simulink model "gm_sampleModel61556_pp_34_1_sub"  (R2023b)
settings: Solver=VariableStepAuto  StartTime=0.0  StopTime=10.0  RelTol=1e-3
libraries: simulink x34
(part 1 of 2)
settings Model: Creator=CW  LastModifiedBy=CW
settings OptimizationCC: BlockReduction=off  ConditionallyExecuteInputs=off
settings DebuggingCC: ArtificialAlgebraicLoopMsg=none  InheritedTsInSrcMsg=none

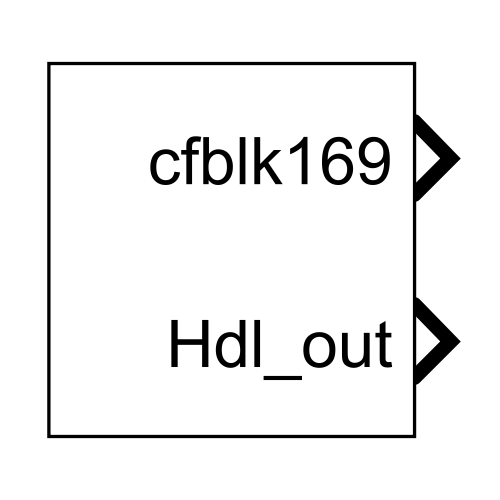
[thumbnail: Simulink's stored preview of the top-level diagram]
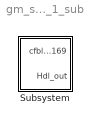
== system gm_sampleModel61556_pp_34_1_sub ==
  Subsystem : Subsystem

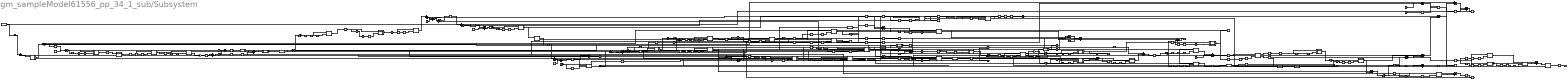
== system gm_sampleModel61556_pp_34_1_sub/Subsystem ==
  Reshape{,1..5} (6 alike) : Reshape
  cfblk1 : Subsystem  mask(Compare To Zero){relop=<=, OutDataTypeStr=uint8, ZeroCross=on}
      mask prompts: relop "Simulink:masks:Operator_MP"; OutDataTypeStr "Simulink:masks:OutputDataType_MP"; ZeroCross "Simulink:masks:EnableZerocrossingDetection_MP"
      mask help: Simulink:masks:CompareToZero_MD
      mask init:
      | OutDataTypeStr = 'uint8';
      | ZeroCross = 'on';
      | blkName = 'sampleModel61556_pp_34_1_sub/Subsystem/cfblk1';
      | relop = '<=';
      | setValue = 'fixdt(0, 8)';
      mask TypeOptions relop: == | ~= | < | <= | >= | >
      mask TypeOptions OutDataTypeStr: Simulink:masks:uint8 | Simulink:masks:boolean
      mask Callback ZeroCross: sl('zeroCrossEnable', gcbh);
      mask Display: disp([relop,' 0'])
  cfblk10 : Subsystem
  cfblk102_inst : Subsystem
  cfblk103 : Subsystem
  cfblk{19,24,26,50,55,57,59,72,104..105,112,115,128,136,138,141,147,158,160} (19 alike) : Sum  OutDataTypeStr=uint8  AccumDataTypeStr=uint8  SampleTime=1
  cfblk{11,30,53,71,81,97,106} (7 alike) : Sum  Inputs=+  OutDataTypeStr=uint8
  cfblk{13,20,22,32,46,82,85,88,107,116,121,134..135,140,154} (15 alike) : Sum  Inputs=+-  OutDataTypeStr=uint8  AccumDataTypeStr=uint8  SampleTime=1
  cfblk{5,15,42,109,123,145..146,162} (8 alike) : Product  Inputs=*/  OutDataTypeStr=uint8  RndMeth=Zero  SaturateOnIntegerOverflow=on  SampleTime=1
  cfblk110 : Subsystem  mask(Real World Value Increment){}
      mask help: Simulink:masks:RealWorldValueIncrement_MD
      mask Display: disp('V++')
  cfblk111 : Subsystem
  cfblk113 : Signum  SampleTime=1
  cfblk{52,80,114,126} (4 alike) : Gain  Gain="fi(0,0,8,7,\"hex\",\"80\")"  ParamDataTypeStr=fixdt(0, 8, 7)  OutDataTypeStr=uint8  SampleTime=1
  cfblk118 : Subsystem
  cfblk119 : Subsystem
  cfblk12 : Subsystem
  cfblk{7,23,25,31,51,63..64,73,87,98,122,142..143,149,152} (15 alike) : MinMax  OutDataTypeStr=uint8
  cfblk{6,41,44,47,60,75,124,132,161,163} (10 alike) : Sum  OutDataTypeStr=uint8  AccumDataTypeStr=uint8  RndMeth=Nearest  SampleTime=1
  cfblk124_const_val : Constant  Value=0  VectorParams1D=off  OutDataTypeStr=uint8  SampleTime=1
  cfblk125 : Subsystem
  cfblk127 : Subsystem
  cfblk129 : Subsystem
  cfblk{17,68,74,99,131,155..156,159} (8 alike) : Abs  SampleTime=1  OutDataTypeStr=uint8  SaturateOnIntegerOverflow=off
  cfblk132_const_val : Constant  Value=0  VectorParams1D=off  OutDataTypeStr=uint8  SampleTime=1
  cfblk133 : Subsystem
  cfblk139 : Subsystem
  cfblk14 : ComplexToRealImag  SampleTime=1
  cfblk144 : Subsystem
  cfblk150 : ComplexToRealImag  SampleTime=1
  cfblk153 : Subsystem
  cfblk157 : Subsystem
  cfblk16 : Subsystem  mask(Real World Value Increment){}
      mask help: Simulink:masks:RealWorldValueIncrement_MD
      mask Display: disp('V++')
  cfblk161_const_val : Constant  Value=0  VectorParams1D=off  OutDataTypeStr=uint8  SampleTime=1
  cfblk163_const_val : Constant  Value=0  VectorParams1D=off  OutDataTypeStr=uint8  SampleTime=1
  cfblk171 : Constant  OutDataTypeStr=uint8  SampleTime=1
  cfblk172 : Constant  OutDataTypeStr=uint8  SampleTime=1
  cfblk173 : Subsystem
  cfblk175 : Subsystem
  cfblk176 : Subsystem
  cfblk177 : Subsystem
  cfblk178 : Subsystem
  cfblk179 : Subsystem
  cfblk180 : Switch  Threshold=double(0)  OutDataTypeStr=uint8  SampleTime=1  SaturateOnIntegerOverflow=off  InputSameDT=off
  cfblk184 : Switch  Threshold=double(0)  OutDataTypeStr=uint8  SampleTime=1  SaturateOnIntegerOverflow=off  InputSameDT=off
  cfblk{186..190,192..197,199..205} (18 alike) : Delay  DelayLength=double(2)  InitialCondition=0  SampleTime=1
  cfblk191 : Subsystem
  cfblk2 : Subsystem  mask(Detect Rise Nonnegative){vinit=double(0), InputProcessing=Elements as channels (sample based), OutDataTypeStr=uint8}
      mask prompts: vinit "Simulink:masks:InitialCondition_MP"; InputProcessing "Simulink:masks:InputProcessing_MP"; OutDataTypeStr "Simulink:masks:OutputDataType_MP"
      mask help: Simulink:masks:DetectRiseNonnegative_MD
      mask init:
      | InputProcessing = 'Elements as channels (sample based)';
      | OutDataTypeStr = 'uint8';
      | vinit = double(0);
      mask TypeOptions InputProcessing: Simulink:masks:ColumnsAsChannelsFrameBased | Simulink:masks:ElementsAsChannelsSampleBased
      mask TypeOptions OutDataTypeStr: Simulink:masks:uint8 | Simulink:masks:boolean
      mask Display: fprintf('U >= 0\n&  NOT\nU/z >= 0')
  cfblk{206..207,209..210,213..215} (7 alike) : DataTypeConversion  OutDataTypeStr=fixdt(0,8,0)
  cfblk208 : Subsystem
  cfblk21 : Subsystem
  cfblk211 : Subsystem
  cfblk212 : Subsystem
  cfblk3 : Subsystem
  cfblk35 : Subsystem
  cfblk36 : Subsystem
  cfblk37 : Subsystem
  cfblk38 : Subsystem  mask(Real World Value Increment){}
      mask help: Simulink:masks:RealWorldValueIncrement_MD
      mask Display: disp('V++')
  cfblk39 : ComplexToRealImag  SampleTime=1
  cfblk4 : Subsystem
  cfblk41_const_val : Constant  Value=0  VectorParams1D=off  OutDataTypeStr=uint8  SampleTime=1
  cfblk43_inst : Subsystem
  cfblk44_const_val : Constant  Value=0  VectorParams1D=off  OutDataTypeStr=uint8  SampleTime=1
  cfblk47_const_val : Constant  Value=0  VectorParams1D=off  OutDataTypeStr=uint8  SampleTime=1
  cfblk49 : Subsystem
  cfblk54 : Subsystem
  cfblk60_const_val : Constant  Value=0  VectorParams1D=off  OutDataTypeStr=uint8  SampleTime=1
  cfblk61_const_val : Constant  Value=double(0)  VectorParams1D=off  OutDataTypeStr=double  SampleTime=1
  cfblk62 : Signum  SampleTime=1
  cfblk65 : Subsystem
  cfblk66 : Subsystem  mask(Real World Value Increment){}
      mask help: Simulink:masks:RealWorldValueIncrement_MD
      mask Display: disp('V++')
  cfblk67 : Subsystem  mask(Real World Value Increment){}
      mask help: Simulink:masks:RealWorldValueIncrement_MD
      mask Display: disp('V++')
  cfblk6_const_val : Constant  Value=0  VectorParams1D=off  OutDataTypeStr=uint8  SampleTime=1
  cfblk70_inst : Subsystem
  cfblk75_const_val : Constant  Value=0  VectorParams1D=off  OutDataTypeStr=uint8  SampleTime=1
  cfblk78 : Subsystem
  cfblk8 : Subsystem
  cfblk83 : Subsystem
  cfblk84_inst : Subsystem
  cfblk86 : Subsystem
  cfblk9 : Subsystem
  cfblk90_inst : Subsystem
  cfblk91 : Subsystem
  cfblk93_inst : Subsystem
  cfblk96 : Subsystem
  compare{,1..3,6,9,14..15,21..24,26,28,32} (15 alike) : simulink/Logic and Bit Operations/Compare To Constant  relop=>=  const=255  OutDataTypeStr=boolean
  compare{4..5,7..8,10..13,16..20,25,27,29..31,33} (19 alike) : simulink/Logic and Bit Operations/Compare To Constant  relop=>=  const=0  OutDataTypeStr=boolean
  emi_{6,22,30,38,46,55,63,79,87,96,104,112,120,128,136,144,152,160,168,176,184,192,200,225,233,241,249,257,266,274,282,298,306,314} (34 alike) : DataTypeConversion  OutDataTypeStr=fixdt(0,8,0)
  emi_{7,31,39,88,105,113,121,129,153,177,226,234,283,299,307} (15 alike) : Delay  DelayLength=double(2)  InitialCondition=255  SampleTime=1
  emi_{23,47,56,64,80,97,137,145,161,169,185,193,201,242,250,258,267,275,315} (19 alike) : Delay  DelayLength=double(2)  InitialCondition=0  SampleTime=1
  cfblk169 : Outport  OutDataTypeStr=uint8  SampleTime=1  InitialOutput=[0]  VectorParamsAs1DForOutWhenUnconnected=off
  Hdl_out : Outport  Port=2  OutDataTypeStr=uint8  SampleTime=1
  wires:
  cfblk1/1(y) -> Reshape1/1
  cfblk10/1(emi_2) -> cfblk66/1(u)
  cfblk102_inst/1(out1) -> cfblk180/2
  cfblk103/1(emi_18) -> cfblk15/1
  cfblk104/1 -> emi_113/1, cfblk144/1(emi_107)
  cfblk105/1 -> cfblk32/2, cfblk115/2
  cfblk106/1 -> emi_121/1, cfblk191/1(emi_115)
  cfblk107/1 -> cfblk31/1
  cfblk109/1 -> cfblk93_inst/1(in1)
  cfblk11/1 -> Reshape5/1
  cfblk110/1(y) -> cfblk46/1, cfblk197/1
  cfblk111/1(emi_26) -> cfblk82/1, cfblk67/1(u)
  cfblk112/1 -> cfblk206/1
  cfblk113/1 -> cfblk126/1
  cfblk114/1 -> cfblk214/1
  cfblk115/1 -> cfblk80/1
  cfblk116/1 -> cfblk41/1
  cfblk118/1(emi_42) -> cfblk5/2, cfblk71/1
  cfblk119/1(emi_50) -> cfblk158/2
  cfblk119/2(emi_51) -> cfblk6/1
  cfblk12/1(emi_59) -> cfblk150/1, cfblk134/2
  cfblk121/1 -> cfblk109/2, cfblk11/1
  cfblk122/1 -> cfblk154/2
  cfblk123/1 -> cfblk81/1
  cfblk124/1 -> cfblk107/1, emi_315/1, cfblk96/1(emi_309)
  cfblk125/1(emi_75) -> cfblk209/1
  cfblk126/1 -> cfblk134/1
  cfblk127/1(emi_83) -> cfblk25/1
  cfblk128/1 -> cfblk121/1
  cfblk129/1(emi_91) -> cfblk210/1
  cfblk129/2(emi_92) -> cfblk14/1
  cfblk13/1 -> emi_226/1, cfblk49/1(emi_219)
  cfblk131/1 -> cfblk16/1(u)
  cfblk132/1 -> emi_234/1, cfblk212/1(emi_228)
  cfblk133/1(emi_148) -> emi_299/1, cfblk9/1(emi_293), cfblk23/1
  cfblk134/1 -> cfblk26/1
  cfblk135/1 -> cfblk116/2
  cfblk136/1 -> cfblk147/1
  cfblk138/1 -> cfblk154/1
  cfblk139/1(emi_100) -> cfblk138/2, cfblk179/1(In1)
  cfblk14/1 -> cfblk160/2
  cfblk14/2 -> cfblk175/1(In1)
  cfblk140/1 -> cfblk138/1, emi_169/1, cfblk3/1(emi_163)
  cfblk141/1 -> cfblk24/1, cfblk200/1
  cfblk142/1 -> cfblk20/1
  cfblk143/1 -> emi_161/1, cfblk211/1(emi_155)
  cfblk144/1(emi_108) -> cfblk55/1
  cfblk145/1 -> emi_275/1, emi_193/1, cfblk83/1(emi_269), cfblk37/1(emi_187)
  cfblk146/1 -> cfblk141/1, cfblk102_inst/1(in1)
  cfblk147/1 -> cfblk202/1
  Reshape/1 -> cfblk84_inst/1(in1)
  cfblk149/1 -> cfblk104/1
  cfblk15/1 -> cfblk99/1
  cfblk150/1 -> cfblk64/1
  cfblk150/2 -> Reshape3/1, cfblk97/1
  cfblk152/1 -> cfblk57/1
  cfblk153/1(emi_124) -> cfblk194/1, cfblk193/1
  cfblk154/1 -> cfblk135/1, cfblk51/1
  cfblk155/1 -> cfblk57/2
  cfblk156/1 -> emi_88/1, cfblk127/1(emi_82)
  cfblk157/1(emi_34) -> emi_283/1, cfblk86/1(emi_277)
  cfblk158/1 -> cfblk142/1
  cfblk159/1 -> cfblk195/1, cfblk42/2
  cfblk16/1(y) -> cfblk155/1
  cfblk160/1 -> cfblk105/2, cfblk145/1
  cfblk161/1 -> cfblk146/2
  cfblk162/1 -> emi_105/1, cfblk139/1(emi_99)
  cfblk163/1 -> cfblk173/1(In1)
  cfblk17/1 -> emi_47/1, cfblk118/1(emi_41)
  cfblk171/1 -> cfblk7/1
  cfblk172/1 -> cfblk26/2
  cfblk173/1(Out1) -> cfblk178/1(In1), cfblk42/1
  cfblk175/1(Out1) -> cfblk2/1(U)
  cfblk176/1(Out1) -> cfblk113/1, cfblk190/1
  cfblk177/1(Out1) -> cfblk75/1
  cfblk178/1(Out1) -> cfblk46/2
  cfblk179/1(Out1) -> cfblk149/1
  cfblk180/1 -> cfblk85/1
  cfblk184/1 -> cfblk136/1, cfblk53/1
  cfblk186/1 -> cfblk109/1
  cfblk187/1 -> cfblk135/2
  cfblk188/1 -> cfblk59/1
  cfblk189/1 -> cfblk128/1
  cfblk19/1 -> cfblk73/1
  cfblk190/1 -> cfblk162/2
  cfblk191/1(emi_116) -> cfblk140/2
  cfblk192/1 -> cfblk93_inst/2(in2)
  cfblk193/1 -> cfblk184/1
  cfblk194/1 -> cfblk180/3
  cfblk195/1 -> cfblk121/2
  cfblk196/1 -> cfblk19/1
  cfblk197/1 -> cfblk184/3
  cfblk199/1 -> cfblk22/2
  cfblk2/1(Y) -> cfblk180/1
  cfblk20/1 -> cfblk177/1(In1)
  cfblk200/1 -> cfblk84_inst/2(in2)
  cfblk201/1 -> cfblk146/1
  cfblk202/1 -> cfblk1/1(u)
  cfblk203/1 -> cfblk85/2
  cfblk204/1 -> cfblk88/1
  cfblk205/1 -> cfblk43_inst/2(in2)
  cfblk206/1 -> cfblk199/1
  cfblk207/1 -> cfblk112/1
  cfblk208/1(emi_132) -> cfblk112/2
  cfblk209/1 -> emi_201/1, cfblk205/1, cfblk4/1(emi_195)
  cfblk21/1(emi_140) -> cfblk59/2, cfblk131/1
  cfblk210/1 -> emi_80/1, cfblk125/1(emi_74)
  cfblk211/1(emi_156) -> cfblk88/2
  cfblk212/1(emi_229) -> cfblk143/1
  cfblk213/1 -> cfblk44/1, cfblk207/1
  cfblk214/1 -> cfblk72/1
  cfblk215/1 -> cfblk72/2
  cfblk22/1 -> cfblk43_inst/1(in1)
  cfblk23/1 -> emi_31/1, cfblk111/1(emi_25)
  cfblk24/1 -> cfblk60/1
  cfblk25/1 -> emi_39/1, cfblk157/1(emi_33)
  cfblk26/1 -> cfblk70_inst/2(in2)
  cfblk3/1(emi_164) -> cfblk19/2, cfblk13/2
  cfblk30/1 -> cfblk20/2
  cfblk31/1 -> cfblk39/1, emi_137/1, cfblk208/1(emi_131)
  cfblk32/1 -> cfblk136/2, cfblk201/1
  Reshape1/1 -> cfblk22/1
  cfblk35/1(emi_172) -> cfblk70_inst/1(in1), cfblk15/2
  cfblk36/1(emi_180) -> emi_267/1, cfblk8/1(emi_260)
  cfblk37/1(emi_188) -> emi_242/1, cfblk54/1(emi_236)
  cfblk38/1(y) -> cfblk163/1
  cfblk39/1 -> cfblk160/1
  cfblk39/2 -> cfblk152/1
  cfblk4/1(emi_196) -> cfblk107/2, cfblk105/1
  cfblk41/1 -> cfblk158/1, Hdl_out/1
  cfblk42/1 -> cfblk196/1
  cfblk43_inst/1(out1) -> cfblk184/2
  cfblk44/1 -> Reshape4/1
  cfblk46/1 -> cfblk156/1
  cfblk47/1 -> cfblk123/1
  cfblk49/1(emi_220) -> cfblk62/1
  cfblk49/2(emi_221) -> cfblk52/1
  cfblk5/1 -> cfblk55/2, emi_129/1, cfblk153/1(emi_123)
  cfblk50/1 -> cfblk90_inst/1(in1)
  cfblk51/1 -> emi_153/1, cfblk133/1(emi_147)
  cfblk52/1 -> cfblk17/1
  cfblk53/1 -> cfblk124/1
  cfblk54/1(emi_237) -> cfblk50/2
  cfblk55/1 -> cfblk186/1
  cfblk57/1 -> cfblk87/1
  Reshape2/1 -> cfblk169/1
  cfblk59/1 -> cfblk161/1
  cfblk6/1 -> cfblk82/2, emi_97/1, cfblk129/1(emi_90)
  cfblk60/1 -> emi_307/1, cfblk91/1(emi_301)
  cfblk62/1 -> cfblk176/1(In1), cfblk106/1
  cfblk63/1 -> cfblk204/1
  cfblk64/1 -> cfblk32/1, cfblk104/2, emi_250/1, cfblk65/1(emi_244)
  cfblk65/1(emi_245) -> cfblk90_inst/2(in2), emi_23/1, cfblk103/1(emi_17), cfblk30/1
  cfblk66/1(y) -> cfblk159/1
  cfblk67/1(y) -> cfblk110/1(u)
  cfblk68/1 -> emi_56/1, emi_145/1, cfblk21/1(emi_139), cfblk119/1(emi_49), cfblk5/1
  cfblk7/1 -> cfblk123/2
  cfblk70_inst/1(out1) -> cfblk188/1
  cfblk71/1 -> cfblk192/1
  cfblk72/1 -> cfblk213/1
  cfblk73/1 -> cfblk68/1
  cfblk74/1 -> emi_177/1, cfblk35/1(emi_171)
  cfblk75/1 -> cfblk74/1
  cfblk78/1(emi_253) -> cfblk215/1
  Reshape3/1 -> cfblk203/1
  cfblk8/1(emi_261) -> cfblk140/1
  cfblk8/2(emi_262) -> cfblk114/1
  cfblk80/1 -> cfblk132/1, cfblk162/1
  cfblk81/1 -> cfblk147/2
  cfblk82/1 -> cfblk24/2, emi_7/1, cfblk10/1(emi_1)
  cfblk83/1(emi_270) -> cfblk50/1
  cfblk84_inst/1(out1) -> emi_185/1, cfblk36/1(emi_179)
  cfblk85/1 -> cfblk128/2
  cfblk86/1(emi_278) -> cfblk116/1
  cfblk87/1 -> cfblk145/2
  cfblk88/1 -> emi_64/1, emi_258/1, cfblk78/1(emi_252), cfblk12/1(emi_58)
  cfblk9/1(emi_294) -> cfblk189/1
  cfblk90_inst/1(out1) -> Reshape2/1
  cfblk91/1(emi_302) -> cfblk13/1
  Reshape4/1 -> cfblk141/2, cfblk38/1(u)
  cfblk93_inst/1(out1) -> cfblk115/1
  Reshape5/1 -> cfblk47/1
  cfblk96/1(emi_310) -> Reshape/1
  cfblk97/1 -> cfblk63/1
  cfblk98/1 -> cfblk102_inst/2(in2)
  cfblk99/1 -> cfblk187/1
  emi_104/1 -> compare/1
  emi_105/1 -> emi_104/1
  emi_112/1 -> compare1/1
  emi_113/1 -> emi_112/1
  emi_120/1 -> compare2/1
  emi_121/1 -> emi_120/1
  emi_128/1 -> compare3/1
  emi_129/1 -> emi_128/1
  emi_136/1 -> compare4/1
  emi_137/1 -> emi_136/1
  emi_144/1 -> compare5/1
  emi_145/1 -> emi_144/1
  emi_152/1 -> compare6/1
  emi_153/1 -> emi_152/1
  emi_160/1 -> compare7/1
  emi_161/1 -> emi_160/1
  emi_168/1 -> compare8/1
  emi_169/1 -> emi_168/1
  emi_176/1 -> compare9/1
  emi_177/1 -> emi_176/1
  emi_184/1 -> compare10/1
  emi_185/1 -> emi_184/1
  emi_192/1 -> compare11/1
  emi_193/1 -> emi_192/1
  emi_200/1 -> compare12/1
  emi_201/1 -> emi_200/1
  emi_22/1 -> compare13/1
  emi_225/1 -> compare14/1
  emi_226/1 -> emi_225/1
  emi_23/1 -> emi_22/1
  emi_233/1 -> compare15/1
  emi_234/1 -> emi_233/1
  emi_241/1 -> compare16/1
  emi_242/1 -> emi_241/1
  emi_249/1 -> compare17/1
  emi_250/1 -> emi_249/1
  emi_257/1 -> compare18/1
  emi_258/1 -> emi_257/1
  emi_266/1 -> compare19/1
  emi_267/1 -> emi_266/1
  emi_274/1 -> compare20/1
  emi_275/1 -> emi_274/1
  emi_282/1 -> compare21/1
  emi_283/1 -> emi_282/1
  emi_298/1 -> compare23/1
  emi_299/1 -> emi_298/1
  emi_30/1 -> compare22/1
  emi_306/1 -> compare24/1
  emi_307/1 -> emi_306/1
  emi_31/1 -> emi_30/1
  emi_314/1 -> compare25/1
  emi_315/1 -> emi_314/1
  emi_38/1 -> compare26/1
  emi_39/1 -> emi_38/1
  emi_46/1 -> compare27/1
  emi_47/1 -> emi_46/1
  emi_55/1 -> compare29/1
  emi_56/1 -> emi_55/1
  emi_6/1 -> compare28/1
  emi_63/1 -> compare30/1
  emi_64/1 -> emi_63/1
  emi_7/1 -> emi_6/1
  emi_79/1 -> compare31/1
  emi_80/1 -> emi_79/1
  emi_87/1 -> compare32/1
  emi_88/1 -> emi_87/1
  emi_96/1 -> compare33/1
  emi_97/1 -> emi_96/1
  cfblk124_const_val/1 -> cfblk124/2
  cfblk132_const_val/1 -> cfblk132/2
  cfblk161_const_val/1 -> cfblk161/2
  cfblk163_const_val/1 -> cfblk163/2
  cfblk41_const_val/1 -> cfblk41/2
  cfblk44_const_val/1 -> cfblk44/2
  cfblk47_const_val/1 -> cfblk47/2
  cfblk6_const_val/1 -> cfblk6/2
  cfblk60_const_val/1 -> cfblk60/2
  cfblk61_const_val/1 -> cfblk98/1, cfblk122/1
  cfblk75_const_val/1 -> cfblk75/2
  compare/1 -> cfblk139/2(Action Port)
  compare1/1 -> cfblk144/2(Action Port)
  compare2/1 -> cfblk191/2(Action Port)
  compare3/1 -> cfblk153/2(Action Port)
  compare4/1 -> cfblk208/2(Action Port)
  compare5/1 -> cfblk21/2(Action Port)
  compare6/1 -> cfblk133/2(Action Port)
  compare7/1 -> cfblk211/2(Action Port)
  compare8/1 -> cfblk3/2(Action Port)
  compare9/1 -> cfblk35/2(Action Port)
  compare10/1 -> cfblk36/2(Action Port)
  compare11/1 -> cfblk37/2(Action Port)
  compare12/1 -> cfblk4/2(Action Port)
  compare13/1 -> cfblk103/2(Action Port)
  compare14/1 -> cfblk49/2(Action Port)
  compare15/1 -> cfblk212/2(Action Port)
  compare16/1 -> cfblk54/2(Action Port)
  compare17/1 -> cfblk65/2(Action Port)
  compare18/1 -> cfblk78/2(Action Port)
  compare19/1 -> cfblk8/2(Action Port)
  compare20/1 -> cfblk83/2(Action Port)
  compare21/1 -> cfblk86/2(Action Port)
  compare22/1 -> cfblk111/2(Action Port)
  compare23/1 -> cfblk9/2(Action Port)
  compare24/1 -> cfblk91/2(Action Port)
  compare25/1 -> cfblk96/2(Action Port)
  compare26/1 -> cfblk157/2(Action Port)
  compare27/1 -> cfblk118/2(Action Port)
  compare28/1 -> cfblk10/2(Action Port)
  compare29/1 -> cfblk119/2(Action Port)
  compare30/1 -> cfblk12/2(Action Port)
  compare31/1 -> cfblk125/2(Action Port)
  compare32/1 -> cfblk127/2(Action Port)
  compare33/1 -> cfblk129/2(Action Port)

== system gm_sampleModel61556_pp_34_1_sub/Subsystem/cfblk1 ==
  u : Inport  OutDataTypeStr=uint8  SampleTime=1
  Compare : RelationalOperator  Operator=<=  OutDataTypeStr=fixdt(0, 8)
  Constant : Constant  DisableCoverage=on  Value=0  OutDataTypeStr=Inherit: Inherit via back propagation  SampleTime=-1  PreserveConstantTs=on
  y : Outport  SampleTime=1
  wires:
  u/1 -> Compare/1
  Compare/1 -> y/1
  Constant/1 -> Compare/2

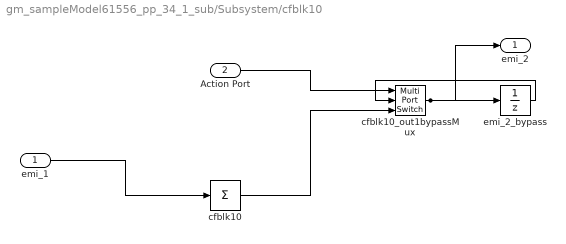
== system gm_sampleModel61556_pp_34_1_sub/Subsystem/cfblk10 ==
  emi_1 : Inport  OutDataTypeStr=uint8  PortDimensions=1  SampleTime=1
  Action Port : Inport  Port=2  OutDataTypeStr=boolean  SampleTime=1
  cfblk10 : Sum  Inputs=+
  cfblk10_out1bypassMux : MultiPortSwitch  DataPortOrder=Zero-based contiguous  Inputs=2  zeroidx=on  OutDataTypeStr=uint8  SampleTime=1  SaturateOnIntegerOverflow=off  InputSameDT=off
  emi_2_bypass : UnitDelay  InitialCondition="fi(0,0,8,0,\"hex\",\"00\")"  SampleTime=1
  emi_2 : Outport  SampleTime=1  InitialOutput=0
  wires:
  Action Port/1 -> cfblk10_out1bypassMux/1
  emi_1/1 -> cfblk10/1
  cfblk10/1 -> cfblk10_out1bypassMux/3
  cfblk10_out1bypassMux/1 -> emi_2_bypass/1, emi_2/1
  emi_2_bypass/1 -> cfblk10_out1bypassMux/2

== system gm_sampleModel61556_pp_34_1_sub/Subsystem/cfblk102_inst ==
  in1 : Inport  OutDataTypeStr=uint8  SampleTime=1
  in2 : Inport  Port=2  OutDataTypeStr=uint8  SampleTime=1
  mul_cfblk102_dotp_mulcomp : Product  Inputs=**  OutDataTypeStr=uint8  SampleTime=1
  out1 : Outport  OutDataTypeStr=uint8  SampleTime=1
  wires:
  in1/1 -> mul_cfblk102_dotp_mulcomp/1
  in2/1 -> mul_cfblk102_dotp_mulcomp/2
  mul_cfblk102_dotp_mulcomp/1 -> out1/1

== system gm_sampleModel61556_pp_34_1_sub/Subsystem/cfblk103 ==
  emi_17 : Inport  OutDataTypeStr=uint8  PortDimensions=1  SampleTime=1
  Action Port : Inport  Port=2  OutDataTypeStr=boolean  SampleTime=1
  cfblk103 : Abs  SampleTime=1  OutDataTypeStr=uint8  SaturateOnIntegerOverflow=off
  cfblk103_out1bypassMux : MultiPortSwitch  DataPortOrder=Zero-based contiguous  Inputs=2  zeroidx=on  OutDataTypeStr=uint8  SampleTime=1  SaturateOnIntegerOverflow=off  InputSameDT=off
  emi_18_bypass : UnitDelay  InitialCondition="fi(0,0,8,0,\"hex\",\"00\")"  SampleTime=1
  emi_18 : Outport  SampleTime=1  InitialOutput=0
  wires:
  Action Port/1 -> cfblk103_out1bypassMux/1
  emi_17/1 -> cfblk103/1
  cfblk103/1 -> cfblk103_out1bypassMux/3
  cfblk103_out1bypassMux/1 -> emi_18_bypass/1, emi_18/1
  emi_18_bypass/1 -> cfblk103_out1bypassMux/2

== system gm_sampleModel61556_pp_34_1_sub/Subsystem/cfblk110 ==
  u : Inport  OutDataTypeStr=uint8  SampleTime=1
  FixPt Constant : Constant  DisableCoverage=on  OutDataTypeStr=Inherit: Inherit via back propagation  SampleTime=-1
  FixPt Data Type Duplicate : DataTypeDuplicate  DisableCoverage=on  NumInputPorts=3
  FixPt Sum1 : Sum  OutDataTypeStr=Inherit: Inherit via back propagation  InputSameDT=on  LockScale=on
  y : Outport  SampleTime=1
  wires:
  u/1 -> FixPt Sum1/1, FixPt Data Type Duplicate/2
  FixPt Constant/1 -> FixPt Sum1/2, FixPt Data Type Duplicate/3
  FixPt Sum1/1 -> FixPt Data Type Duplicate/1, y/1

== system gm_sampleModel61556_pp_34_1_sub/Subsystem/cfblk111 ==
  emi_25 : Inport  OutDataTypeStr=uint8  PortDimensions=1  SampleTime=1
  Action Port : Inport  Port=2  OutDataTypeStr=boolean  SampleTime=1
  cfblk111 : Subsystem  mask(Real World Value Increment){}
      mask help: Simulink:masks:RealWorldValueIncrement_MD
      mask Display: disp('V++')
  cfblk111_out1bypassMux : MultiPortSwitch  DataPortOrder=Zero-based contiguous  Inputs=2  zeroidx=on  OutDataTypeStr=uint8  SampleTime=1  SaturateOnIntegerOverflow=off  InputSameDT=off
  emi_26_bypass : UnitDelay  InitialCondition="fi(0,0,8,0,\"hex\",\"00\")"  SampleTime=1
  emi_26 : Outport  SampleTime=1  InitialOutput=0
  wires:
  Action Port/1 -> cfblk111_out1bypassMux/1
  emi_25/1 -> cfblk111/1(u)
  cfblk111/1(y) -> cfblk111_out1bypassMux/3
  cfblk111_out1bypassMux/1 -> emi_26_bypass/1, emi_26/1
  emi_26_bypass/1 -> cfblk111_out1bypassMux/2

== system gm_sampleModel61556_pp_34_1_sub/Subsystem/cfblk118 ==
  emi_41 : Inport  OutDataTypeStr=uint8  PortDimensions=1  SampleTime=1
  Action Port : Inport  Port=2  OutDataTypeStr=boolean  SampleTime=1
  cfblk118 : MinMax
  cfblk118_out1bypassMux : MultiPortSwitch  DataPortOrder=Zero-based contiguous  Inputs=2  zeroidx=on  OutDataTypeStr=uint8  SampleTime=1  SaturateOnIntegerOverflow=off  InputSameDT=off
  emi_42_bypass : UnitDelay  InitialCondition="fi(0,0,8,0,\"hex\",\"00\")"  SampleTime=1
  emi_42 : Outport  SampleTime=1  InitialOutput=0
  wires:
  Action Port/1 -> cfblk118_out1bypassMux/1
  emi_41/1 -> cfblk118/1
  cfblk118/1 -> cfblk118_out1bypassMux/3
  cfblk118_out1bypassMux/1 -> emi_42_bypass/1, emi_42/1
  emi_42_bypass/1 -> cfblk118_out1bypassMux/2

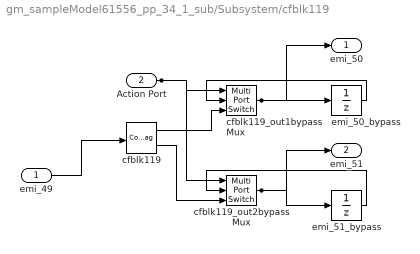
== system gm_sampleModel61556_pp_34_1_sub/Subsystem/cfblk119 ==
  emi_49 : Inport  OutDataTypeStr=uint8  PortDimensions=1  SampleTime=1
  Action Port : Inport  Port=2  OutDataTypeStr=boolean  SampleTime=1
  cfblk119 : ComplexToRealImag  SampleTime=1
  cfblk119_out1bypassMux : MultiPortSwitch  DataPortOrder=Zero-based contiguous  Inputs=2  zeroidx=on  OutDataTypeStr=uint8  SampleTime=1  SaturateOnIntegerOverflow=off  InputSameDT=off
  cfblk119_out2bypassMux : MultiPortSwitch  DataPortOrder=Zero-based contiguous  Inputs=2  zeroidx=on  OutDataTypeStr=uint8  SampleTime=1  SaturateOnIntegerOverflow=off  InputSameDT=off
  emi_50_bypass : UnitDelay  InitialCondition="fi(0,0,8,0,\"hex\",\"00\")"  SampleTime=1
  emi_51_bypass : UnitDelay  InitialCondition="fi(0,0,8,0,\"hex\",\"00\")"  SampleTime=1
  emi_50 : Outport  SampleTime=1  InitialOutput=0
  emi_51 : Outport  Port=2  SampleTime=1  InitialOutput=0
  wires:
  Action Port/1 -> cfblk119_out2bypassMux/1, cfblk119_out1bypassMux/1
  emi_49/1 -> cfblk119/1
  cfblk119/1 -> cfblk119_out1bypassMux/3
  cfblk119/2 -> cfblk119_out2bypassMux/3
  cfblk119_out1bypassMux/1 -> emi_50_bypass/1, emi_50/1
  emi_50_bypass/1 -> cfblk119_out1bypassMux/2
  cfblk119_out2bypassMux/1 -> emi_51_bypass/1, emi_51/1
  emi_51_bypass/1 -> cfblk119_out2bypassMux/2

== system gm_sampleModel61556_pp_34_1_sub/Subsystem/cfblk12 ==
  emi_58 : Inport  OutDataTypeStr=uint8  PortDimensions=1  SampleTime=1
  Action Port : Inport  Port=2  OutDataTypeStr=boolean  SampleTime=1
  cfblk12 : Sum  Inputs=+
  cfblk12_out1bypassMux : MultiPortSwitch  DataPortOrder=Zero-based contiguous  Inputs=2  zeroidx=on  OutDataTypeStr=uint8  SampleTime=1  SaturateOnIntegerOverflow=off  InputSameDT=off
  emi_59_bypass : UnitDelay  InitialCondition="fi(0,0,8,0,\"hex\",\"00\")"  SampleTime=1
  emi_59 : Outport  SampleTime=1  InitialOutput=0
  wires:
  Action Port/1 -> cfblk12_out1bypassMux/1
  emi_58/1 -> cfblk12/1
  cfblk12/1 -> cfblk12_out1bypassMux/3
  cfblk12_out1bypassMux/1 -> emi_59_bypass/1, emi_59/1
  emi_59_bypass/1 -> cfblk12_out1bypassMux/2

== system gm_sampleModel61556_pp_34_1_sub/Subsystem/cfblk125 ==
  emi_74 : Inport  OutDataTypeStr=uint8  PortDimensions=1  SampleTime=1
  Action Port : Inport  Port=2  OutDataTypeStr=boolean  SampleTime=1
  cfblk125 : MinMax
  cfblk125_out1bypassMux : MultiPortSwitch  DataPortOrder=Zero-based contiguous  Inputs=2  zeroidx=on  OutDataTypeStr=uint8  SampleTime=1  SaturateOnIntegerOverflow=off  InputSameDT=off
  emi_75_bypass : UnitDelay  InitialCondition="fi(0,0,8,0,\"hex\",\"00\")"  SampleTime=1
  emi_75 : Outport  SampleTime=1  InitialOutput=0
  wires:
  Action Port/1 -> cfblk125_out1bypassMux/1
  emi_74/1 -> cfblk125/1
  cfblk125/1 -> cfblk125_out1bypassMux/3
  cfblk125_out1bypassMux/1 -> emi_75_bypass/1, emi_75/1
  emi_75_bypass/1 -> cfblk125_out1bypassMux/2

== system gm_sampleModel61556_pp_34_1_sub/Subsystem/cfblk127 ==
  emi_82 : Inport  OutDataTypeStr=uint8  PortDimensions=1  SampleTime=1
  Action Port : Inport  Port=2  OutDataTypeStr=boolean  SampleTime=1
  cfblk127 : MinMax
  cfblk127_out1bypassMux : MultiPortSwitch  DataPortOrder=Zero-based contiguous  Inputs=2  zeroidx=on  OutDataTypeStr=uint8  SampleTime=1  SaturateOnIntegerOverflow=off  InputSameDT=off
  emi_83_bypass : UnitDelay  InitialCondition="fi(0,0,8,0,\"hex\",\"00\")"  SampleTime=1
  emi_83 : Outport  SampleTime=1  InitialOutput=0
  wires:
  Action Port/1 -> cfblk127_out1bypassMux/1
  emi_82/1 -> cfblk127/1
  cfblk127/1 -> cfblk127_out1bypassMux/3
  cfblk127_out1bypassMux/1 -> emi_83_bypass/1, emi_83/1
  emi_83_bypass/1 -> cfblk127_out1bypassMux/2

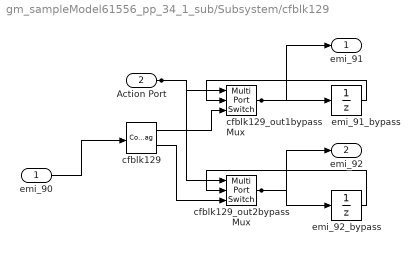
== system gm_sampleModel61556_pp_34_1_sub/Subsystem/cfblk129 ==
  emi_90 : Inport  OutDataTypeStr=uint8  PortDimensions=1  SampleTime=1
  Action Port : Inport  Port=2  OutDataTypeStr=boolean  SampleTime=1
  cfblk129 : ComplexToRealImag  SampleTime=1
  cfblk129_out1bypassMux : MultiPortSwitch  DataPortOrder=Zero-based contiguous  Inputs=2  zeroidx=on  OutDataTypeStr=uint8  SampleTime=1  SaturateOnIntegerOverflow=off  InputSameDT=off
  cfblk129_out2bypassMux : MultiPortSwitch  DataPortOrder=Zero-based contiguous  Inputs=2  zeroidx=on  OutDataTypeStr=uint8  SampleTime=1  SaturateOnIntegerOverflow=off  InputSameDT=off
  emi_91_bypass : UnitDelay  InitialCondition="fi(0,0,8,0,\"hex\",\"00\")"  SampleTime=1
  emi_92_bypass : UnitDelay  InitialCondition="fi(0,0,8,0,\"hex\",\"00\")"  SampleTime=1
  emi_91 : Outport  SampleTime=1  InitialOutput=0
  emi_92 : Outport  Port=2  SampleTime=1  InitialOutput=0
  wires:
  Action Port/1 -> cfblk129_out2bypassMux/1, cfblk129_out1bypassMux/1
  emi_90/1 -> cfblk129/1
  cfblk129/1 -> cfblk129_out1bypassMux/3
  cfblk129/2 -> cfblk129_out2bypassMux/3
  cfblk129_out1bypassMux/1 -> emi_91_bypass/1, emi_91/1
  emi_91_bypass/1 -> cfblk129_out1bypassMux/2
  cfblk129_out2bypassMux/1 -> emi_92_bypass/1, emi_92/1
  emi_92_bypass/1 -> cfblk129_out2bypassMux/2

== system gm_sampleModel61556_pp_34_1_sub/Subsystem/cfblk133 ==
  emi_147 : Inport  OutDataTypeStr=uint8  PortDimensions=1  SampleTime=1
  Action Port : Inport  Port=2  OutDataTypeStr=boolean  SampleTime=1
  Reshape : Reshape
  cfblk133_out1bypassMux : MultiPortSwitch  DataPortOrder=Zero-based contiguous  Inputs=2  zeroidx=on  OutDataTypeStr=uint8  SampleTime=1  SaturateOnIntegerOverflow=off  InputSameDT=off
  emi_148_bypass : UnitDelay  InitialCondition="fi(0,0,8,0,\"hex\",\"00\")"  SampleTime=1
  emi_148 : Outport  SampleTime=1  InitialOutput=0
  wires:
  Action Port/1 -> cfblk133_out1bypassMux/1
  emi_147/1 -> Reshape/1
  Reshape/1 -> cfblk133_out1bypassMux/3
  cfblk133_out1bypassMux/1 -> emi_148_bypass/1, emi_148/1
  emi_148_bypass/1 -> cfblk133_out1bypassMux/2

== system gm_sampleModel61556_pp_34_1_sub/Subsystem/cfblk139 ==
  emi_99 : Inport  OutDataTypeStr=uint8  PortDimensions=1  SampleTime=1
  Action Port : Inport  Port=2  OutDataTypeStr=boolean  SampleTime=1
  Reshape : Reshape
  cfblk139_out1bypassMux : MultiPortSwitch  DataPortOrder=Zero-based contiguous  Inputs=2  zeroidx=on  OutDataTypeStr=uint8  SampleTime=1  SaturateOnIntegerOverflow=off  InputSameDT=off
  emi_100_bypass : UnitDelay  InitialCondition="fi(0,0,8,0,\"hex\",\"00\")"  SampleTime=1
  emi_100 : Outport  SampleTime=1  InitialOutput=0
  wires:
  Action Port/1 -> cfblk139_out1bypassMux/1
  emi_99/1 -> Reshape/1
  Reshape/1 -> cfblk139_out1bypassMux/3
  cfblk139_out1bypassMux/1 -> emi_100_bypass/1, emi_100/1
  emi_100_bypass/1 -> cfblk139_out1bypassMux/2

== system gm_sampleModel61556_pp_34_1_sub/Subsystem/cfblk144 ==
  emi_107 : Inport  OutDataTypeStr=uint8  PortDimensions=1  SampleTime=1
  Action Port : Inport  Port=2  OutDataTypeStr=boolean  SampleTime=1
  cfblk144 : Abs  SampleTime=1  OutDataTypeStr=uint8  SaturateOnIntegerOverflow=off
  cfblk144_out1bypassMux : MultiPortSwitch  DataPortOrder=Zero-based contiguous  Inputs=2  zeroidx=on  OutDataTypeStr=uint8  SampleTime=1  SaturateOnIntegerOverflow=off  InputSameDT=off
  emi_108_bypass : UnitDelay  InitialCondition="fi(0,0,8,0,\"hex\",\"00\")"  SampleTime=1
  emi_108 : Outport  SampleTime=1  InitialOutput=0
  wires:
  Action Port/1 -> cfblk144_out1bypassMux/1
  emi_107/1 -> cfblk144/1
  cfblk144/1 -> cfblk144_out1bypassMux/3
  cfblk144_out1bypassMux/1 -> emi_108_bypass/1, emi_108/1
  emi_108_bypass/1 -> cfblk144_out1bypassMux/2

== system gm_sampleModel61556_pp_34_1_sub/Subsystem/cfblk153 ==
  emi_123 : Inport  OutDataTypeStr=uint8  PortDimensions=1  SampleTime=1
  Action Port : Inport  Port=2  OutDataTypeStr=boolean  SampleTime=1
  cfblk153 : Subsystem  mask(Real World Value Increment){}
      mask help: Simulink:masks:RealWorldValueIncrement_MD
      mask Display: disp('V++')
  cfblk153_out1bypassMux : MultiPortSwitch  DataPortOrder=Zero-based contiguous  Inputs=2  zeroidx=on  OutDataTypeStr=uint8  SampleTime=1  SaturateOnIntegerOverflow=off  InputSameDT=off
  emi_124_bypass : UnitDelay  InitialCondition="fi(0,0,8,0,\"hex\",\"00\")"  SampleTime=1
  emi_124 : Outport  SampleTime=1  InitialOutput=0
  wires:
  Action Port/1 -> cfblk153_out1bypassMux/1
  emi_123/1 -> cfblk153/1(u)
  cfblk153/1(y) -> cfblk153_out1bypassMux/3
  cfblk153_out1bypassMux/1 -> emi_124_bypass/1, emi_124/1
  emi_124_bypass/1 -> cfblk153_out1bypassMux/2

== system gm_sampleModel61556_pp_34_1_sub/Subsystem/cfblk157 ==
  emi_33 : Inport  OutDataTypeStr=uint8  PortDimensions=1  SampleTime=1
  Action Port : Inport  Port=2  OutDataTypeStr=boolean  SampleTime=1
  cfblk157 : Abs  SampleTime=1  OutDataTypeStr=uint8  SaturateOnIntegerOverflow=off
  cfblk157_out1bypassMux : MultiPortSwitch  DataPortOrder=Zero-based contiguous  Inputs=2  zeroidx=on  OutDataTypeStr=uint8  SampleTime=1  SaturateOnIntegerOverflow=off  InputSameDT=off
  emi_34_bypass : UnitDelay  InitialCondition="fi(0,0,8,0,\"hex\",\"00\")"  SampleTime=1
  emi_34 : Outport  SampleTime=1  InitialOutput=0
  wires:
  Action Port/1 -> cfblk157_out1bypassMux/1
  emi_33/1 -> cfblk157/1
  cfblk157/1 -> cfblk157_out1bypassMux/3
  cfblk157_out1bypassMux/1 -> emi_34_bypass/1, emi_34/1
  emi_34_bypass/1 -> cfblk157_out1bypassMux/2

== system gm_sampleModel61556_pp_34_1_sub/Subsystem/cfblk16 ==
  u : Inport  OutDataTypeStr=uint8  SampleTime=1
  FixPt Constant : Constant  DisableCoverage=on  OutDataTypeStr=Inherit: Inherit via back propagation  SampleTime=-1
  FixPt Data Type Duplicate : DataTypeDuplicate  DisableCoverage=on  NumInputPorts=3
  FixPt Sum1 : Sum  OutDataTypeStr=Inherit: Inherit via back propagation  InputSameDT=on  LockScale=on
  y : Outport  SampleTime=1
  wires:
  u/1 -> FixPt Sum1/1, FixPt Data Type Duplicate/2
  FixPt Constant/1 -> FixPt Sum1/2, FixPt Data Type Duplicate/3
  FixPt Sum1/1 -> FixPt Data Type Duplicate/1, y/1

== system gm_sampleModel61556_pp_34_1_sub/Subsystem/cfblk173 ==
  In1 : Inport  OutDataTypeStr=uint8  PortDimensions=1  SampleTime=1
  Out1 : Outport  SampleTime=1  InitialOutput=[0]
  wires:
  In1/1 -> Out1/1

== system gm_sampleModel61556_pp_34_1_sub/Subsystem/cfblk175 ==
  In1 : Inport  OutDataTypeStr=uint8  PortDimensions=1  SampleTime=1
  Out1 : Outport  SampleTime=1  InitialOutput=[0]
  wires:
  In1/1 -> Out1/1

== system gm_sampleModel61556_pp_34_1_sub/Subsystem/cfblk176 ==
  In1 : Inport  OutDataTypeStr=uint8  PortDimensions=1  SampleTime=1
  Out1 : Outport  SampleTime=1  InitialOutput=[0]
  wires:
  In1/1 -> Out1/1

== system gm_sampleModel61556_pp_34_1_sub/Subsystem/cfblk177 ==
  In1 : Inport  OutDataTypeStr=uint8  PortDimensions=1  SampleTime=1
  Out1 : Outport  SampleTime=1  InitialOutput=[0]
  wires:
  In1/1 -> Out1/1

== system gm_sampleModel61556_pp_34_1_sub/Subsystem/cfblk178 ==
  In1 : Inport  OutDataTypeStr=uint8  PortDimensions=1  SampleTime=1
  Out1 : Outport  SampleTime=1  InitialOutput=[0]
  wires:
  In1/1 -> Out1/1

== system gm_sampleModel61556_pp_34_1_sub/Subsystem/cfblk179 ==
  In1 : Inport  OutDataTypeStr=uint8  PortDimensions=1  SampleTime=1
  Out1 : Outport  SampleTime=1  InitialOutput=[0]
  wires:
  In1/1 -> Out1/1

== system gm_sampleModel61556_pp_34_1_sub/Subsystem/cfblk191 ==
  emi_115 : Inport  OutDataTypeStr=uint8  PortDimensions=1  SampleTime=1
  Action Port : Inport  Port=2  OutDataTypeStr=boolean  SampleTime=1
  cfblk191 : Subsystem
      settings: MinAlgLoopOccurrences=on
  emi_116 : Outport  SampleTime=1  InitialOutput=0
  wires:
  Action Port/1 -> cfblk191/Enable
  emi_115/1 -> cfblk191/1(in0)
  cfblk191/1(out0) -> emi_116/1

== system gm_sampleModel61556_pp_34_1_sub/Subsystem/cfblk2 ==
  note: U(k)
  note: Edge
  U : Inport  OutDataTypeStr=uint8  SampleTime=1
  Delay Input1 : UnitDelay  Description=Store in Global RAM  DisableCoverage=on  InitialCondition=vinit  SampleTime=-1  HasFrameUpgradeWarning=on
  FixPt Relational Operator : RelationalOperator  Operator=>  OutDataTypeStr=fixdt(0, 8)  ZeroCross=off  InputSameDT=off
  Nonnegative : Subsystem  mask(Compare To Zero){relop=>=, OutDataTypeStr=boolean, ZeroCross=off}
      mask prompts: relop "Simulink:masks:Operator_MP"; OutDataTypeStr "Simulink:masks:OutputDataType_MP"; ZeroCross "Simulink:masks:EnableZerocrossingDetection_MP"
      mask help: Simulink:masks:CompareToZero_MD
      mask init:
      | OutDataTypeStr = 'boolean';
      | ZeroCross = 'off';
      | blkName = 'sampleModel61556_pp_34_1_sub/Subsystem/cfblk2/Nonnegative';
      | relop = '>=';
      | setValue = 'boolean';
      mask TypeOptions relop: == | ~= | < | <= | >= | >
      mask TypeOptions OutDataTypeStr: Simulink:masks:uint8 | Simulink:masks:boolean
      mask Callback ZeroCross: sl('zeroCrossEnable', gcbh);
      mask Display: disp([relop,' 0'])
  Y : Outport  SampleTime=1
  wires:
  U/1 -> Nonnegative/1(u)
  Delay Input1/1 -> FixPt Relational Operator/2
  FixPt Relational Operator/1 -> Y/1
  Nonnegative/1(y) -> FixPt Relational Operator/1, Delay Input1/1

== system gm_sampleModel61556_pp_34_1_sub/Subsystem/cfblk208 ==
  emi_131 : Inport  OutDataTypeStr=uint8  PortDimensions=1  SampleTime=1
  Action Port : Inport  Port=2  OutDataTypeStr=boolean  SampleTime=1
  cfblk208 : DataTypeConversion  OutDataTypeStr=fixdt(0,8,0)
  cfblk208_out1bypassMux : MultiPortSwitch  DataPortOrder=Zero-based contiguous  Inputs=2  zeroidx=on  OutDataTypeStr=uint8  SampleTime=1  SaturateOnIntegerOverflow=off  InputSameDT=off
  emi_132_bypass : UnitDelay  InitialCondition="fi(0,0,8,0,\"hex\",\"00\")"  SampleTime=1
  emi_132 : Outport  SampleTime=1  InitialOutput=0
  wires:
  Action Port/1 -> cfblk208_out1bypassMux/1
  emi_131/1 -> cfblk208/1
  cfblk208/1 -> cfblk208_out1bypassMux/3
  cfblk208_out1bypassMux/1 -> emi_132_bypass/1, emi_132/1
  emi_132_bypass/1 -> cfblk208_out1bypassMux/2

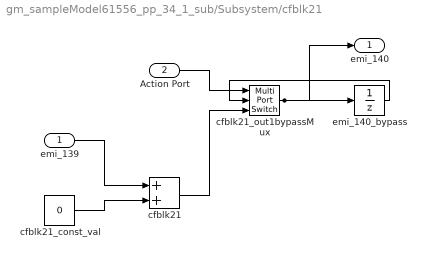
== system gm_sampleModel61556_pp_34_1_sub/Subsystem/cfblk21 ==
  emi_139 : Inport  OutDataTypeStr=uint8  PortDimensions=1  SampleTime=1
  Action Port : Inport  Port=2  OutDataTypeStr=boolean  SampleTime=1
  cfblk21 : Sum  OutDataTypeStr=uint8  AccumDataTypeStr=uint8  RndMeth=Nearest  SampleTime=1
  cfblk21_const_val : Constant  Value=0  VectorParams1D=off  OutDataTypeStr=uint8  SampleTime=1
  cfblk21_out1bypassMux : MultiPortSwitch  DataPortOrder=Zero-based contiguous  Inputs=2  zeroidx=on  OutDataTypeStr=uint8  SampleTime=1  SaturateOnIntegerOverflow=off  InputSameDT=off
  emi_140_bypass : UnitDelay  InitialCondition="fi(0,0,8,0,\"hex\",\"00\")"  SampleTime=1
  emi_140 : Outport  SampleTime=1  InitialOutput=0
  wires:
  Action Port/1 -> cfblk21_out1bypassMux/1
  emi_139/1 -> cfblk21/1
  cfblk21/1 -> cfblk21_out1bypassMux/3
  cfblk21_out1bypassMux/1 -> emi_140_bypass/1, emi_140/1
  emi_140_bypass/1 -> cfblk21_out1bypassMux/2
  cfblk21_const_val/1 -> cfblk21/2

== system gm_sampleModel61556_pp_34_1_sub/Subsystem/cfblk211 ==
  emi_155 : Inport  OutDataTypeStr=uint8  PortDimensions=1  SampleTime=1
  Action Port : Inport  Port=2  OutDataTypeStr=boolean  SampleTime=1
  cfblk211 : DataTypeConversion  OutDataTypeStr=fixdt(0,8,0)
  cfblk211_out1bypassMux : MultiPortSwitch  DataPortOrder=Zero-based contiguous  Inputs=2  zeroidx=on  OutDataTypeStr=uint8  SampleTime=1  SaturateOnIntegerOverflow=off  InputSameDT=off
  emi_156_bypass : UnitDelay  InitialCondition="fi(0,0,8,0,\"hex\",\"00\")"  SampleTime=1
  emi_156 : Outport  SampleTime=1  InitialOutput=0
  wires:
  Action Port/1 -> cfblk211_out1bypassMux/1
  emi_155/1 -> cfblk211/1
  cfblk211/1 -> cfblk211_out1bypassMux/3
  cfblk211_out1bypassMux/1 -> emi_156_bypass/1, emi_156/1
  emi_156_bypass/1 -> cfblk211_out1bypassMux/2

== system gm_sampleModel61556_pp_34_1_sub/Subsystem/cfblk212 ==
  emi_228 : Inport  OutDataTypeStr=uint8  PortDimensions=1  SampleTime=1
  Action Port : Inport  Port=2  OutDataTypeStr=boolean  SampleTime=1
  cfblk212 : DataTypeConversion  OutDataTypeStr=fixdt(0,8,0)
  cfblk212_out1bypassMux : MultiPortSwitch  DataPortOrder=Zero-based contiguous  Inputs=2  zeroidx=on  OutDataTypeStr=uint8  SampleTime=1  SaturateOnIntegerOverflow=off  InputSameDT=off
  emi_229_bypass : UnitDelay  InitialCondition="fi(0,0,8,0,\"hex\",\"00\")"  SampleTime=1
  emi_229 : Outport  SampleTime=1  InitialOutput=0
  wires:
  Action Port/1 -> cfblk212_out1bypassMux/1
  emi_228/1 -> cfblk212/1
  cfblk212/1 -> cfblk212_out1bypassMux/3
  cfblk212_out1bypassMux/1 -> emi_229_bypass/1, emi_229/1
  emi_229_bypass/1 -> cfblk212_out1bypassMux/2

== system gm_sampleModel61556_pp_34_1_sub/Subsystem/cfblk3 ==
  emi_163 : Inport  OutDataTypeStr=uint8  PortDimensions=1  SampleTime=1
  Action Port : Inport  Port=2  OutDataTypeStr=boolean  SampleTime=1
  cfblk3 : Constant  Value=0  OutDataTypeStr=uint8  SampleTime=1
  cfblk3_out1bypassMux : MultiPortSwitch  DataPortOrder=Zero-based contiguous  Inputs=2  zeroidx=on  OutDataTypeStr=uint8  SampleTime=1  SaturateOnIntegerOverflow=off  InputSameDT=off
  emi_164_bypass : UnitDelay  InitialCondition="fi(0,0,8,0,\"hex\",\"00\")"  SampleTime=1
  emi_164 : Outport  SampleTime=1  InitialOutput=0
  wires:
  Action Port/1 -> cfblk3_out1bypassMux/1
  cfblk3/1 -> cfblk3_out1bypassMux/3
  cfblk3_out1bypassMux/1 -> emi_164_bypass/1, emi_164/1
  emi_164_bypass/1 -> cfblk3_out1bypassMux/2

== system gm_sampleModel61556_pp_34_1_sub/Subsystem/cfblk35 ==
  emi_171 : Inport  OutDataTypeStr=uint8  PortDimensions=1  SampleTime=1
  Action Port : Inport  Port=2  OutDataTypeStr=boolean  SampleTime=1
  cfblk35 : Abs  SampleTime=1  OutDataTypeStr=uint8  SaturateOnIntegerOverflow=off
  cfblk35_out1bypassMux : MultiPortSwitch  DataPortOrder=Zero-based contiguous  Inputs=2  zeroidx=on  OutDataTypeStr=uint8  SampleTime=1  SaturateOnIntegerOverflow=off  InputSameDT=off
  emi_172_bypass : UnitDelay  InitialCondition="fi(0,0,8,0,\"hex\",\"00\")"  SampleTime=1
  emi_172 : Outport  SampleTime=1  InitialOutput=0
  wires:
  Action Port/1 -> cfblk35_out1bypassMux/1
  emi_171/1 -> cfblk35/1
  cfblk35/1 -> cfblk35_out1bypassMux/3
  cfblk35_out1bypassMux/1 -> emi_172_bypass/1, emi_172/1
  emi_172_bypass/1 -> cfblk35_out1bypassMux/2

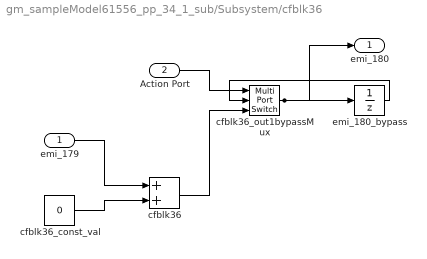
== system gm_sampleModel61556_pp_34_1_sub/Subsystem/cfblk36 ==
  emi_179 : Inport  OutDataTypeStr=uint8  PortDimensions=1  SampleTime=1
  Action Port : Inport  Port=2  OutDataTypeStr=boolean  SampleTime=1
  cfblk36 : Sum  OutDataTypeStr=uint8  AccumDataTypeStr=uint8  RndMeth=Nearest  SampleTime=1
  cfblk36_const_val : Constant  Value=0  VectorParams1D=off  OutDataTypeStr=uint8  SampleTime=1
  cfblk36_out1bypassMux : MultiPortSwitch  DataPortOrder=Zero-based contiguous  Inputs=2  zeroidx=on  OutDataTypeStr=uint8  SampleTime=1  SaturateOnIntegerOverflow=off  InputSameDT=off
  emi_180_bypass : UnitDelay  InitialCondition="fi(0,0,8,0,\"hex\",\"00\")"  SampleTime=1
  emi_180 : Outport  SampleTime=1  InitialOutput=0
  wires:
  Action Port/1 -> cfblk36_out1bypassMux/1
  emi_179/1 -> cfblk36/1
  cfblk36/1 -> cfblk36_out1bypassMux/3
  cfblk36_out1bypassMux/1 -> emi_180_bypass/1, emi_180/1
  emi_180_bypass/1 -> cfblk36_out1bypassMux/2
  cfblk36_const_val/1 -> cfblk36/2

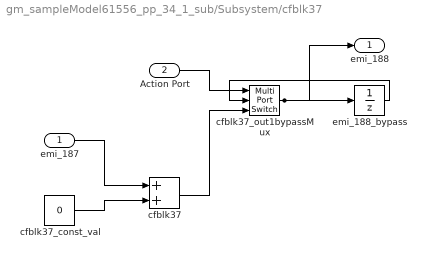
== system gm_sampleModel61556_pp_34_1_sub/Subsystem/cfblk37 ==
  emi_187 : Inport  OutDataTypeStr=uint8  PortDimensions=1  SampleTime=1
  Action Port : Inport  Port=2  OutDataTypeStr=boolean  SampleTime=1
  cfblk37 : Sum  OutDataTypeStr=uint8  AccumDataTypeStr=uint8  RndMeth=Nearest  SampleTime=1
  cfblk37_const_val : Constant  Value=0  VectorParams1D=off  OutDataTypeStr=uint8  SampleTime=1
  cfblk37_out1bypassMux : MultiPortSwitch  DataPortOrder=Zero-based contiguous  Inputs=2  zeroidx=on  OutDataTypeStr=uint8  SampleTime=1  SaturateOnIntegerOverflow=off  InputSameDT=off
  emi_188_bypass : UnitDelay  InitialCondition="fi(0,0,8,0,\"hex\",\"00\")"  SampleTime=1
  emi_188 : Outport  SampleTime=1  InitialOutput=0
  wires:
  Action Port/1 -> cfblk37_out1bypassMux/1
  emi_187/1 -> cfblk37/1
  cfblk37/1 -> cfblk37_out1bypassMux/3
  cfblk37_out1bypassMux/1 -> emi_188_bypass/1, emi_188/1
  emi_188_bypass/1 -> cfblk37_out1bypassMux/2
  cfblk37_const_val/1 -> cfblk37/2

== system gm_sampleModel61556_pp_34_1_sub/Subsystem/cfblk38 ==
  u : Inport  OutDataTypeStr=uint8  SampleTime=1
  FixPt Constant : Constant  DisableCoverage=on  OutDataTypeStr=Inherit: Inherit via back propagation  SampleTime=-1
  FixPt Data Type Duplicate : DataTypeDuplicate  DisableCoverage=on  NumInputPorts=3
  FixPt Sum1 : Sum  OutDataTypeStr=Inherit: Inherit via back propagation  InputSameDT=on  LockScale=on
  y : Outport  SampleTime=1
  wires:
  u/1 -> FixPt Sum1/1, FixPt Data Type Duplicate/2
  FixPt Constant/1 -> FixPt Sum1/2, FixPt Data Type Duplicate/3
  FixPt Sum1/1 -> FixPt Data Type Duplicate/1, y/1

== system gm_sampleModel61556_pp_34_1_sub/Subsystem/cfblk4 ==
  emi_195 : Inport  OutDataTypeStr=uint8  PortDimensions=1  SampleTime=1
  Action Port : Inport  Port=2  OutDataTypeStr=boolean  SampleTime=1
  cfblk4 : Subsystem  mask(Detect Rise Positive){vinit=double(0), InputProcessing=Elements as channels (sample based), OutDataTypeStr=uint8}
      mask prompts: vinit "Simulink:masks:InitialCondition_MP"; InputProcessing "Simulink:masks:InputProcessing_MP"; OutDataTypeStr "Simulink:masks:OutputDataType_MP"
      mask help: Simulink:masks:DetectRisePositive_MD
      mask TypeOptions InputProcessing: Simulink:masks:ColumnsAsChannelsFrameBased | Simulink:masks:ElementsAsChannelsSampleBased
      mask TypeOptions OutDataTypeStr: Simulink:masks:uint8 | Simulink:masks:boolean
      mask Display: fprintf('U > 0\n&  NOT\nU/z > 0')
  cfblk4_out1bypassMux : MultiPortSwitch  DataPortOrder=Zero-based contiguous  Inputs=2  zeroidx=on  OutDataTypeStr=uint8  SampleTime=1  SaturateOnIntegerOverflow=off  InputSameDT=off
  emi_196_bypass : UnitDelay  InitialCondition="fi(0,0,8,0,\"hex\",\"00\")"  SampleTime=1
  emi_196 : Outport  SampleTime=1  InitialOutput=0
  wires:
  Action Port/1 -> cfblk4_out1bypassMux/1, cfblk4/2(Action Port_out2)
  emi_195/1 -> cfblk4/1(U)
  cfblk4/1(Y) -> cfblk4_out1bypassMux/3
  cfblk4_out1bypassMux/1 -> emi_196_bypass/1, emi_196/1
  emi_196_bypass/1 -> cfblk4_out1bypassMux/2

== system gm_sampleModel61556_pp_34_1_sub/Subsystem/cfblk43_inst ==
  in1 : Inport  OutDataTypeStr=uint8  SampleTime=1
  in2 : Inport  Port=2  OutDataTypeStr=uint8  SampleTime=1
  mul_cfblk43_dotp_mulcomp : Product  Inputs=**  OutDataTypeStr=uint8  SampleTime=1
  out1 : Outport  OutDataTypeStr=uint8  SampleTime=1
  wires:
  in1/1 -> mul_cfblk43_dotp_mulcomp/1
  in2/1 -> mul_cfblk43_dotp_mulcomp/2
  mul_cfblk43_dotp_mulcomp/1 -> out1/1

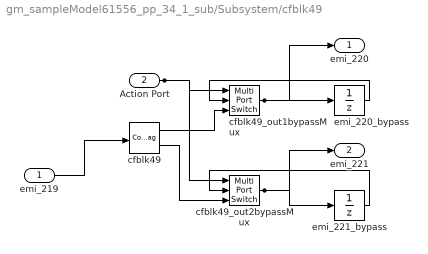
== system gm_sampleModel61556_pp_34_1_sub/Subsystem/cfblk49 ==
  emi_219 : Inport  OutDataTypeStr=uint8  PortDimensions=1  SampleTime=1
  Action Port : Inport  Port=2  OutDataTypeStr=boolean  SampleTime=1
  cfblk49 : ComplexToRealImag  SampleTime=1
  cfblk49_out1bypassMux : MultiPortSwitch  DataPortOrder=Zero-based contiguous  Inputs=2  zeroidx=on  OutDataTypeStr=uint8  SampleTime=1  SaturateOnIntegerOverflow=off  InputSameDT=off
  cfblk49_out2bypassMux : MultiPortSwitch  DataPortOrder=Zero-based contiguous  Inputs=2  zeroidx=on  OutDataTypeStr=uint8  SampleTime=1  SaturateOnIntegerOverflow=off  InputSameDT=off
  emi_220_bypass : UnitDelay  InitialCondition="fi(0,0,8,0,\"hex\",\"00\")"  SampleTime=1
  emi_221_bypass : UnitDelay  InitialCondition="fi(0,0,8,0,\"hex\",\"00\")"  SampleTime=1
  emi_220 : Outport  SampleTime=1  InitialOutput=0
  emi_221 : Outport  Port=2  SampleTime=1  InitialOutput=0
  wires:
  Action Port/1 -> cfblk49_out2bypassMux/1, cfblk49_out1bypassMux/1
  emi_219/1 -> cfblk49/1
  cfblk49/1 -> cfblk49_out1bypassMux/3
  cfblk49/2 -> cfblk49_out2bypassMux/3
  cfblk49_out1bypassMux/1 -> emi_220_bypass/1, emi_220/1
  emi_220_bypass/1 -> cfblk49_out1bypassMux/2
  cfblk49_out2bypassMux/1 -> emi_221_bypass/1, emi_221/1
  emi_221_bypass/1 -> cfblk49_out2bypassMux/2

== system gm_sampleModel61556_pp_34_1_sub/Subsystem/cfblk54 ==
  emi_236 : Inport  OutDataTypeStr=uint8  PortDimensions=1  SampleTime=1
  Action Port : Inport  Port=2  OutDataTypeStr=boolean  SampleTime=1
  cfblk54 : Sum  Inputs=+
  cfblk54_out1bypassMux : MultiPortSwitch  DataPortOrder=Zero-based contiguous  Inputs=2  zeroidx=on  OutDataTypeStr=uint8  SampleTime=1  SaturateOnIntegerOverflow=off  InputSameDT=off
  emi_237_bypass : UnitDelay  InitialCondition="fi(0,0,8,0,\"hex\",\"00\")"  SampleTime=1
  emi_237 : Outport  SampleTime=1  InitialOutput=0
  wires:
  Action Port/1 -> cfblk54_out1bypassMux/1
  emi_236/1 -> cfblk54/1
  cfblk54/1 -> cfblk54_out1bypassMux/3
  cfblk54_out1bypassMux/1 -> emi_237_bypass/1, emi_237/1
  emi_237_bypass/1 -> cfblk54_out1bypassMux/2

== system gm_sampleModel61556_pp_34_1_sub/Subsystem/cfblk65 ==
  emi_244 : Inport  OutDataTypeStr=uint8  PortDimensions=1  SampleTime=1
  Action Port : Inport  Port=2  OutDataTypeStr=boolean  SampleTime=1
  cfblk65 : Sum  Inputs=+
  cfblk65_out1bypassMux : MultiPortSwitch  DataPortOrder=Zero-based contiguous  Inputs=2  zeroidx=on  OutDataTypeStr=uint8  SampleTime=1  SaturateOnIntegerOverflow=off  InputSameDT=off
  emi_245_bypass : UnitDelay  InitialCondition="fi(0,0,8,0,\"hex\",\"00\")"  SampleTime=1
  emi_245 : Outport  SampleTime=1  InitialOutput=0
  wires:
  Action Port/1 -> cfblk65_out1bypassMux/1
  emi_244/1 -> cfblk65/1
  cfblk65/1 -> cfblk65_out1bypassMux/3
  cfblk65_out1bypassMux/1 -> emi_245_bypass/1, emi_245/1
  emi_245_bypass/1 -> cfblk65_out1bypassMux/2

== system gm_sampleModel61556_pp_34_1_sub/Subsystem/cfblk66 ==
  u : Inport  OutDataTypeStr=uint8  SampleTime=1
  FixPt Constant : Constant  DisableCoverage=on  OutDataTypeStr=Inherit: Inherit via back propagation  SampleTime=-1
  FixPt Data Type Duplicate : DataTypeDuplicate  DisableCoverage=on  NumInputPorts=3
  FixPt Sum1 : Sum  OutDataTypeStr=Inherit: Inherit via back propagation  InputSameDT=on  LockScale=on
  y : Outport  SampleTime=1
  wires:
  u/1 -> FixPt Sum1/1, FixPt Data Type Duplicate/2
  FixPt Constant/1 -> FixPt Sum1/2, FixPt Data Type Duplicate/3
  FixPt Sum1/1 -> FixPt Data Type Duplicate/1, y/1

== system gm_sampleModel61556_pp_34_1_sub/Subsystem/cfblk67 ==
  u : Inport  OutDataTypeStr=uint8  SampleTime=1
  FixPt Constant : Constant  DisableCoverage=on  OutDataTypeStr=Inherit: Inherit via back propagation  SampleTime=-1
  FixPt Data Type Duplicate : DataTypeDuplicate  DisableCoverage=on  NumInputPorts=3
  FixPt Sum1 : Sum  OutDataTypeStr=Inherit: Inherit via back propagation  InputSameDT=on  LockScale=on
  y : Outport  SampleTime=1
  wires:
  u/1 -> FixPt Sum1/1, FixPt Data Type Duplicate/2
  FixPt Constant/1 -> FixPt Sum1/2, FixPt Data Type Duplicate/3
  FixPt Sum1/1 -> FixPt Data Type Duplicate/1, y/1

== system gm_sampleModel61556_pp_34_1_sub/Subsystem/cfblk70_inst ==
  in1 : Inport  OutDataTypeStr=uint8  SampleTime=1
  in2 : Inport  Port=2  OutDataTypeStr=uint8  SampleTime=1
  mul_cfblk70_dotp_mulcomp : Product  Inputs=**  OutDataTypeStr=uint8  SampleTime=1
  out1 : Outport  OutDataTypeStr=uint8  SampleTime=1
  wires:
  in1/1 -> mul_cfblk70_dotp_mulcomp/1
  in2/1 -> mul_cfblk70_dotp_mulcomp/2
  mul_cfblk70_dotp_mulcomp/1 -> out1/1
